simulink model "MFCS"  (R2016a)
settings: Solver=VariableStepAuto  StartTime=0.0  StopTime=10  RelTol=1e-3
values from neighbouring files (symbols this model uses):
  A = [ ... (first row only)    [mfcs.m]
  B = [ ... (first row only)    [mfcs.m]
  C = eye(9)    [mfcs.m]
  D = zeros(9,4)    [mfcs.m]
  G1 = [ ... (first row only)    [mfcs.m]
  G2 = [0,0,0,0,0,0,1,0,0 ... (first row only)    [mfcs.m]
  G3 = Baa^(-1)    [mfcs.m]
  G4 = [ ... (first row only)    [mfcs.m]
  G5 = [7,0,0,0 ... (first row only)    [mfcs.m]
  R = [ ... (first row only)    [mfcs.m]
settings Model: Creator=Administrator  LastModifiedBy=Administrator

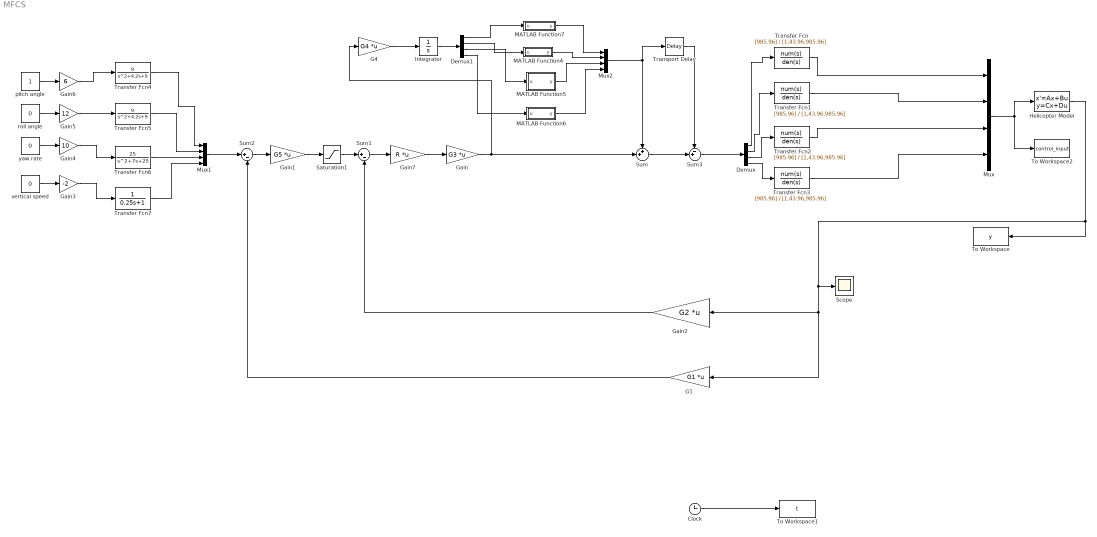
== system MFCS ==
  Clock : Clock
  Demux : Demux
  Demux1 : Demux
  G1 : Gain  Gain=G1  Multiplication=Matrix(K*u)
  G4 : Gain  Gain=G4  Multiplication=Matrix(K*u)
  Gain : Gain  Gain=G3  Multiplication=Matrix(K*u)
  Gain1 : Gain  Gain=G5  Multiplication=Matrix(K*u)
  Gain2 : Gain  Gain=G2  Multiplication=Matrix(K*u)
  Gain3 : Gain  Gain=-2
  Gain4 : Gain  Gain=10
  Gain5 : Gain  Gain=12
  Gain6 : Gain  Gain=6
  Gain7 : Gain  Gain=R  Multiplication=Matrix(K*u)
  "Helicopter Model " : StateSpace  A=A  B=B  C=C  D=D  X0=0
  Integrator : Integrator
  MATLAB Function4 : MATLAB Function  TreatAsAtomicUnit=on
  MATLAB Function5 : MATLAB Function  TreatAsAtomicUnit=on
  MATLAB Function6 : MATLAB Function  TreatAsAtomicUnit=on
  MATLAB Function7 : MATLAB Function  TreatAsAtomicUnit=on
  Mux : Mux
  Mux1 : Mux
  Mux2 : Mux
  Saturation1 : Saturate  UpperLimit=1  LowerLimit=-1
  Scope : Scope
  Sum : Sum  Inputs=++|
  Sum1 : Sum  Inputs=|+-
  Sum2 : Sum  Inputs=|+-
  Sum3 : Sum  Inputs=-+|
  To Workspace : ToWorkspace  VariableName=y  SampleTime=-1
  To Workspace1 : ToWorkspace  VariableName=t  SampleTime=-1
  To Workspace2 : ToWorkspace  VariableName=control_input  SampleTime=-1
  Transfer Fcn{,1..3} (4 alike) : TransferFcn  Numerator=[985.96]  Denominator=[1,43.96,985.96]
  Transfer Fcn4 : TransferFcn  Numerator=[9]  Denominator=[1 4.2 9]
  Transfer Fcn5 : TransferFcn  Numerator=[9]  Denominator=[1 4.2 9]
  Transfer Fcn6 : TransferFcn  Numerator=[25]  Denominator=[1 7 25]
  Transfer Fcn7 : TransferFcn  Denominator=[0.25 1]
  Transport Delay : TransportDelay  DelayTime=0.1
  "pitch angle " : Constant
  roll angle : Constant  Value=0
  vertical speed : Constant  Value=0
  yaw rate : Constant  Value=0
  wires:
  Gain2/1 -> Sum1/2
  G1/1 -> Sum2/2
  "Helicopter Model "/1 -> Scope/1, G1/1, Gain2/1, To Workspace/1
  "pitch angle "/1 -> Gain6/1
  roll angle/1 -> Gain5/1
  yaw rate/1 -> Gain4/1
  vertical speed/1 -> Gain3/1
  Saturation1/1 -> Sum1/1
  Demux/1 -> Transfer Fcn/1
  Demux/2 -> Transfer Fcn1/1
  Demux/3 -> Transfer Fcn2/1
  Demux/4 -> Transfer Fcn3/1
  Gain6/1 -> Transfer Fcn4/1
  Transfer Fcn4/1 -> Mux1/1
  Gain5/1 -> Transfer Fcn5/1
  Transfer Fcn5/1 -> Mux1/2
  Gain4/1 -> Transfer Fcn6/1
  Transfer Fcn6/1 -> Mux1/3
  Gain3/1 -> Transfer Fcn7/1
  Transfer Fcn7/1 -> Mux1/4
  Sum2/1 -> Gain1/1
  Gain1/1 -> Saturation1/1
  Sum1/1 -> Gain7/1
  Mux1/1 -> Sum2/1
  G4/1 -> Integrator/1
  Gain7/1 -> Gain/1
  Gain/1 -> G4/1, Sum/2
  Clock/1 -> To Workspace1/1
  Sum3/1 -> Demux/1
  Sum/1 -> Sum3/2
  Transport Delay/1 -> Sum3/1
  Mux/1 -> "Helicopter Model "/1, To Workspace2/1
  Transfer Fcn/1 -> Mux/1
  Transfer Fcn3/1 -> Mux/4
  Transfer Fcn2/1 -> Mux/3
  Transfer Fcn1/1 -> Mux/2
  Integrator/1 -> Demux1/1
  Demux1/1 -> MATLAB Function7/1(u)
  Demux1/2 -> MATLAB Function4/1(u)
  Demux1/3 -> MATLAB Function5/1(u)
  Demux1/4 -> MATLAB Function6/1(u)
  MATLAB Function7/1(y) -> Mux2/1
  MATLAB Function4/1(y) -> Mux2/2
  MATLAB Function5/1(y) -> Mux2/3
  MATLAB Function6/1(y) -> Mux2/4
  Mux2/1 -> Sum/1, Transport Delay/1

== matlab function MFCS/MATLAB Function4 ==
  data: u input; y output
function y = fcn(u)
%#codegen

if abs(u)>1
    y=0;
else
    y=u;
end

== matlab function MFCS/MATLAB Function5 ==
  data: u input; y output
function y = fcn(u)
%#codegen

if abs(u)>1
    y=0;
else
    y=u;
end

== matlab function MFCS/MATLAB Function6 ==
  data: u input; y output
function y = fcn(u)
%#codegen

if abs(u)>1
    y=0;
else
    y=u;
end

== matlab function MFCS/MATLAB Function7 ==
  data: u input; y output
function y = fcn(u)
%#codegen

if abs(u)>1
    y=0;
else
    y=u;
end
